simulink model "sim_torque_control_PID_PI"  (R2021b)
settings: Solver=ode1  StartTime=0.0  StopTime=60  FixedStep=0.01  RelTol=1e-3
values from neighbouring files (symbols this model uses):
  D = 0.00001    (= 1e-05)    [motor_parameter.m]
  J = 0.0005    [motor_parameter.m]
  Kb = Kt    (= 0.1)    [motor_parameter.m]
  Kt = 0.1    [motor_parameter.m]
  R = 2    [motor_parameter.m]
libraries: simulink_extras x2
settings Model: Creator=DCLab  LastModifiedBy=ASUS

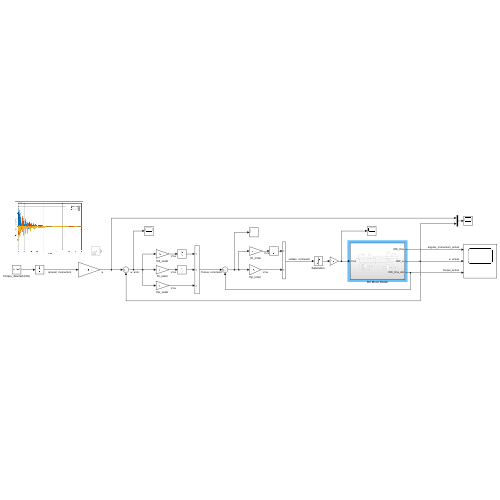
[thumbnail: Simulink's stored preview of the top-level diagram]
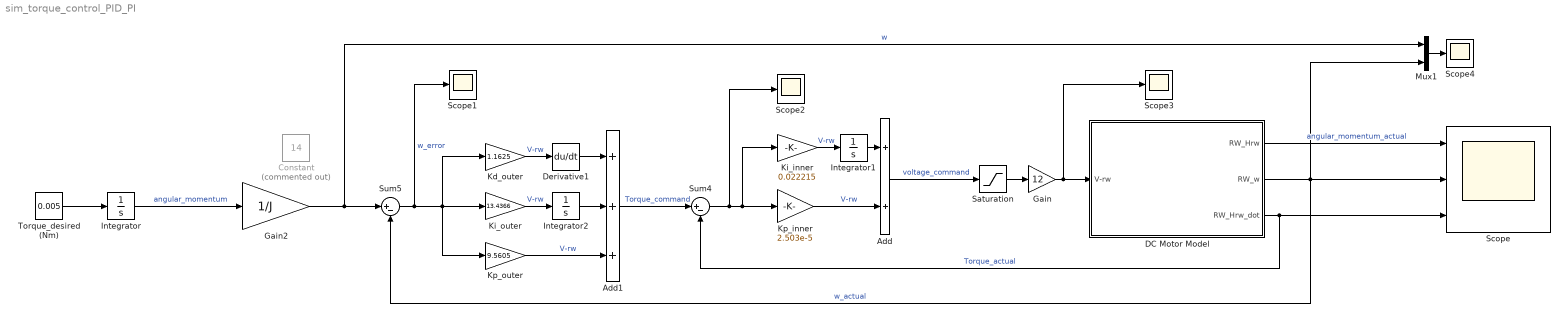
== system sim_torque_control_PID_PI ==
  Add : Sum
  Add1 : Sum  Inputs=+++
  Constant : Constant  Commented=on  Value=14
  DC Motor Model : Subsystem
  Derivative1 : Derivative
  Gain : Gain  Gain=12
  Gain2 : Gain  Gain=1/J
  Integrator : Integrator
  Integrator1 : Integrator
  Integrator2 : Integrator
  Kd_outer : Gain  Gain=1.1625
  Ki_inner : Gain  Gain=0.022215
  Ki_outer : Gain  Gain=13.4366
  Kp_inner : Gain  Gain=2.503e-5
  Kp_outer : Gain  Gain=9.5605
  Mux1 : Mux  Inputs=2
  "Saturation " : Saturate  UpperLimit=20  LowerLimit=-20
  Scope : Scope  NumInputPorts=3
  Scope{1..4} (4 alike) : Scope
  Sum4 : Sum  Inputs=|+-
  Sum5 : Sum  Inputs=|+-
  Torque_desired (Nm) : Constant  Value=0.005
  wires:
  Derivative1/1 -> Add1/1
  Kp_outer/1 -> Add1/3  "V-rw"
  Kd_outer/1 -> Derivative1/1  "V-rw"
  Ki_outer/1 -> Integrator2/1  "V-rw"
  Integrator1/1 -> Add/1
  Kp_inner/1 -> Add/2  "V-rw"
  Gain2/1 -> Mux1/1, Sum5/1  "w"
  Ki_inner/1 -> Integrator1/1  "V-rw"
  DC Motor Model/3(RW_Hrw_dot) -> Scope/3, Sum4/2  "Torque_actual"
  DC Motor Model/2(RW_w) -> Mux1/2, Scope/2, Sum5/2  "w_actual"
  DC Motor Model/1(RW_Hrw) -> Scope/1  "angular_momentum_actual"
  Integrator2/1 -> Add1/2
  Integrator/1 -> Gain2/1  "angular_momentum"
  Add/1 -> "Saturation "/1  "voltage_command"
  Add1/1 -> Sum4/1  "Torque_command"
  Sum5/1 -> Scope1/1, Kp_outer/1, Ki_outer/1, Kd_outer/1  "w_error"
  Sum4/1 -> Scope2/1, Ki_inner/1, Kp_inner/1
  Torque_desired (Nm)/1 -> Integrator/1
  Mux1/1 -> Scope4/1
  "Saturation "/1 -> Gain/1
  Gain/1 -> Scope3/1, DC Motor Model/1(V-rw)

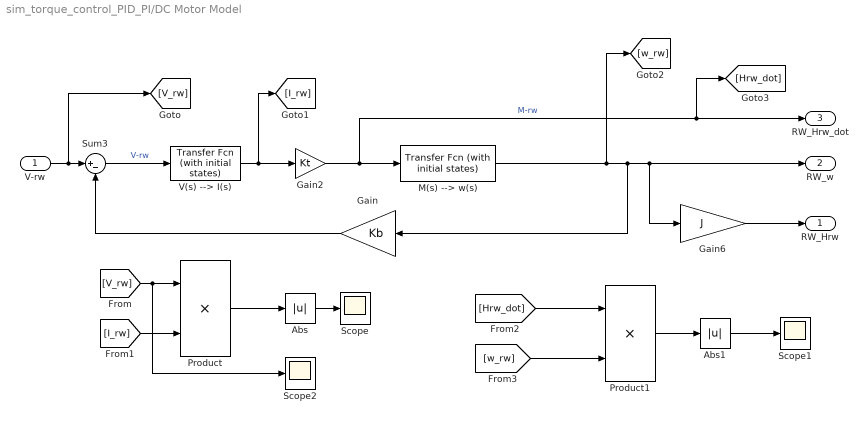
== system sim_torque_control_PID_PI/DC Motor Model ==
  V-rw : Inport
  Abs : Abs
  Abs1 : Abs
  Gain : Gain  Gain=Kb
  Gain2 : Gain  Gain=Kt
  Gain6 : Gain  Gain=J
  M(s) --> w(s) : simulink_extras/Additional Linear/Transfer Fcn (with initial states)  N=[1]  D=[5e-4 D]  X0=0
  Product : Product
  Product1 : Product
  Scope : Scope
  Scope1 : Scope
  Scope2 : Scope
  Sum3 : Sum  Inputs=|+-
  V(s) --> I(s) : simulink_extras/Additional Linear/Transfer Fcn (with initial states)  N=1  D=[R]  X0=0
  RW_Hrw : Outport  VectorParamsAs1DForOutWhenUnconnected=off
  RW_w : Outport  Port=2  VectorParamsAs1DForOutWhenUnconnected=off
  RW_Hrw_dot : Outport  Port=3  VectorParamsAs1DForOutWhenUnconnected=off
  wires:
  V-rw/1 -> [V_rw], Sum3/1
  Gain2/1 -> M(s) --> w(s)/1, [Hrw_dot], RW_Hrw_dot/1  "M-rw"
  Gain6/1 -> RW_Hrw/1
  Gain/1 -> Sum3/2
  Sum3/1 -> V(s) --> I(s)/1  "V-rw"
  V(s) --> I(s)/1 -> [I_rw], Gain2/1
  M(s) --> w(s)/1 -> RW_w/1, Gain6/1, Gain/1, [w_rw]
  [V_rw] -> Scope2/1, Product/1
  [I_rw] -> Product/2
  Product/1 -> Abs/1
  Abs/1 -> Scope/1
  [Hrw_dot] -> Product1/1
  [w_rw] -> Product1/2
  Product1/1 -> Abs1/1
  Abs1/1 -> Scope1/1
